simulink model "rlc2"  (R2020b)
settings: Solver=FixedStepAuto  StartTime=0.0  StopTime=Tk  FixedStep=Ts  RelTol=1e-3
undefined symbols (not defined in the file or in its folder): C, Freq, L, R
settings Model: Creator=Rampage  LastModifiedBy=Rampage

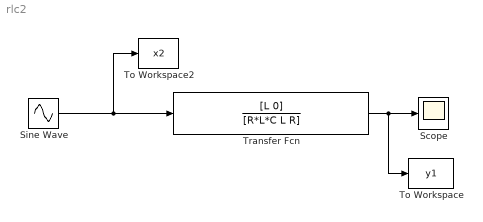
== system rlc2 ==
  Scope : Scope
  Sine Wave : Sin  Frequency=Freq  SampleTime=0
  To Workspace : ToWorkspace  VariableName=y1  SampleTime=-1
  To Workspace2 : ToWorkspace  VariableName=x2  SampleTime=-1
  Transfer Fcn : TransferFcn  Numerator=[L 0]  Denominator=[R*L*C L R]
  wires:
  Sine Wave/1 -> To Workspace2/1, Transfer Fcn/1
  Transfer Fcn/1 -> Scope/1, To Workspace/1
